simulink library "Nibble_Multiplexers_Lib"  (R2023a)
settings: Solver=ode45  StartTime=0.0  StopTime=10.0  RelTol=1e-3  EnableMultiTasking=on
settings Model: Creator=uzivatel  LastModifiedBy=Jozko Mrkvicka
settings SolverCC: AlgebraicLoopSolver=TrustRegion
settings DataIOCC: LimitDataPoints=on  SaveFormat=Array  ReturnWorkspaceOutputs=off
settings OptimizationCC: LifeSpan=inf
settings DebuggingCC: UnderspecifiedInitializationDetection=Classic  MergeDetectMultiDrivingBlocksExec=none  SolverPrmCheckMsg=warning  UnconnectedInputMsg=warning  UnconnectedOutputMsg=warning  UnconnectedLineMsg=warning  StateNameClashWarn=warning  SFUnexpectedBacktrackingDiag=warning  SFNoUnconditionalDefaultTransitionDiag=warning  ArithmeticOperatorsInVariantConditions=warning
settings HardwareCC: ProdBitPerPointer=32  ProdBitPerSizeT=32  ProdBitPerPtrDiffT=32  ProdLargestAtomicFloat=None  ProdIntDivRoundTo=Undefined  ProdEndianess=Unspecified  ProdWordSize=32  ProdHWDeviceType=32-bit Generic
settings ModelReferenceCC: EnableRefExpFcnMdlSchedulingChecks=on  PropagateSignalLabelsOutOfModel=off
settings SFSimCC: SimUseLocalCustomCode=off  CustomCodeUndefinedFunction=UseInterfaceOnly
settings RTWCC: RTWUseLocalCustomCode=off
settings CodeAppCC: StateflowObjectComments=on
settings GRTTargetCC: TargetLangStandard=C89/C90 (ANSI)
settings ConfigComp: CovMetricSettings=dw  CovSaveCumulativeToWorkspaceVar=on  CovSaveSingleToWorkspaceVar=on  CovExternalEMLEnable=off

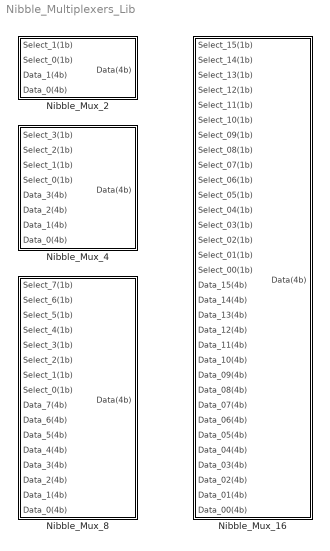
== system Nibble_Multiplexers_Lib ==
  Nibble_Mux_16 : Subsystem
  Nibble_Mux_2 : Subsystem
  Nibble_Mux_4 : Subsystem
  Nibble_Mux_8 : Subsystem

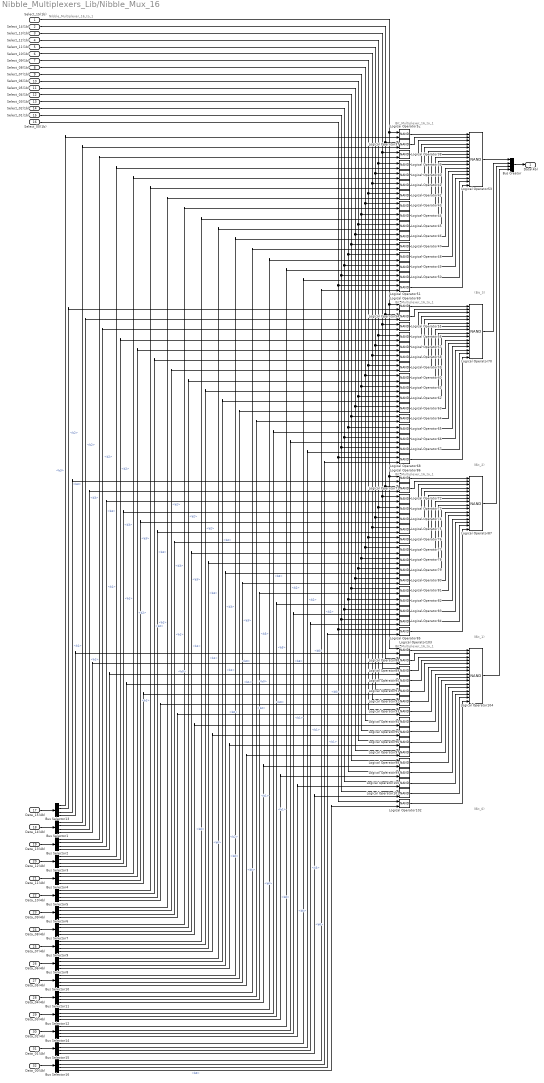
== system Nibble_Multiplexers_Lib/Nibble_Mux_16 ==
  note: (Bit_3)
  note: (Bit_2)
  note: Bit_Multiplexer_16_to_1
  note: (Bit_1)
  note: Bit_Multiplexer_16_to_1
  note: (Bit_0)
  note: Bit_Multiplexer_16_to_1
  note: Bit_Multiplexer_16_to_1
  note: Nibble_Multiplexer_16_to_1
  Select_15(1b) : Inport
  Select_14(1b) : Inport  Port=2
  Select_13(1b) : Inport  Port=3
  Select_12(1b) : Inport  Port=4
  Select_11(1b) : Inport  Port=5
  Select_10(1b) : Inport  Port=6
  Select_09(1b) : Inport  Port=7
  Select_08(1b) : Inport  Port=8
  Select_07(1b) : Inport  Port=9
  Select_06(1b) : Inport  Port=10
  Select_05(1b) : Inport  Port=11
  Select_04(1b) : Inport  Port=12
  Select_03(1b) : Inport  Port=13
  Select_02(1b) : Inport  Port=14
  Select_01(1b) : Inport  Port=15
  Select_00(1b) : Inport  Port=16
  Data_15(4b) : Inport  Port=17
  Data_14(4b) : Inport  Port=18
  Data_13(4b) : Inport  Port=19
  Data_12(4b) : Inport  Port=20
  Data_11(4b) : Inport  Port=21
  Data_10(4b) : Inport  Port=22
  Data_09(4b) : Inport  Port=23
  Data_08(4b) : Inport  Port=24
  Data_07(4b) : Inport  Port=25
  Data_06(4b) : Inport  Port=26
  Data_05(4b) : Inport  Port=27
  Data_04(4b) : Inport  Port=28
  Data_03(4b) : Inport  Port=29
  Data_02(4b) : Inport  Port=30
  Data_01(4b) : Inport  Port=31
  Data_00(4b) : Inport  Port=32
  Bus Creator : BusCreator  Inputs=4
  Bus Selector{1..16} (16 alike) : BusSelector  OutputSignals=b3,b2,b1,b0
  Logical Operator{37..52,54..69,71..86,88..103} (64 alike) : Logic  Operator=NAND  IconShape=distinctive  AllPortsSameDT=off  OutDataTypeStr=boolean
  Logical Operator{53,70,87,104} (4 alike) : Logic  Operator=NAND  Inputs=16  IconShape=distinctive  OutDataTypeStr=boolean
  Data(4b) : Outport
  wires:
  Bus Selector13/1 -> Logical Operator52/2  "<b3>"
  Bus Selector1/1 -> Logical Operator37/2  "<b3>"
  Bus Selector2/1 -> Logical Operator38/2  "<b3>"
  Bus Selector3/1 -> Logical Operator39/2  "<b3>"
  Bus Selector4/1 -> Logical Operator40/2  "<b3>"
  Bus Selector5/1 -> Logical Operator41/2  "<b3>"
  Bus Selector6/1 -> Logical Operator42/2  "<b3>"
  Bus Selector7/1 -> Logical Operator43/2  "<b3>"
  Bus Selector13/2 -> Logical Operator69/2  "<b2>"
  Bus Selector1/2 -> Logical Operator54/2  "<b2>"
  Bus Selector2/2 -> Logical Operator55/2  "<b2>"
  Bus Selector3/2 -> Logical Operator56/2  "<b2>"
  Bus Selector4/2 -> Logical Operator57/2  "<b2>"
  Bus Selector5/2 -> Logical Operator58/2  "<b2>"
  Bus Selector6/2 -> Logical Operator59/2  "<b2>"
  Bus Selector7/2 -> Logical Operator60/2  "<b2>"
  Bus Selector13/3 -> Logical Operator86/2  "<b1>"
  Bus Selector1/3 -> Logical Operator71/2  "<b1>"
  Bus Selector2/3 -> Logical Operator72/2  "<b1>"
  Bus Selector3/3 -> Logical Operator73/2  "<b1>"
  Bus Selector4/3 -> Logical Operator74/2  "<b1>"
  Bus Selector5/3 -> Logical Operator75/2  "<b1>"
  Bus Selector6/3 -> Logical Operator76/2  "<b1>"
  Bus Selector7/3 -> Logical Operator77/2  "<b1>"
  Bus Selector13/4 -> Logical Operator103/2  "<b0>"
  Bus Selector1/4 -> Logical Operator88/2  "<b0>"
  Bus Selector2/4 -> Logical Operator89/2  "<b0>"
  Bus Selector3/4 -> Logical Operator90/2  "<b0>"
  Bus Selector4/4 -> Logical Operator91/2  "<b0>"
  Bus Selector5/4 -> Logical Operator92/2  "<b0>"
  Bus Selector6/4 -> Logical Operator93/2  "<b0>"
  Bus Selector7/4 -> Logical Operator94/2  "<b0>"
  Logical Operator49/1 -> Logical Operator53/14
  Logical Operator43/1 -> Logical Operator53/8
  Logical Operator51/1 -> Logical Operator53/16
  Logical Operator46/1 -> Logical Operator53/11
  Logical Operator50/1 -> Logical Operator53/15
  Logical Operator37/1 -> Logical Operator53/2
  Logical Operator47/1 -> Logical Operator53/12
  Logical Operator39/1 -> Logical Operator53/4
  Logical Operator38/1 -> Logical Operator53/3
  Logical Operator44/1 -> Logical Operator53/9
  Logical Operator45/1 -> Logical Operator53/10
  Logical Operator40/1 -> Logical Operator53/5
  Logical Operator52/1 -> Logical Operator53/1
  Logical Operator42/1 -> Logical Operator53/7
  Logical Operator41/1 -> Logical Operator53/6
  Logical Operator48/1 -> Logical Operator53/13
  Logical Operator66/1 -> Logical Operator70/14
  Logical Operator60/1 -> Logical Operator70/8
  Logical Operator68/1 -> Logical Operator70/16
  Logical Operator63/1 -> Logical Operator70/11
  Logical Operator67/1 -> Logical Operator70/15
  Logical Operator54/1 -> Logical Operator70/2
  Logical Operator64/1 -> Logical Operator70/12
  Logical Operator56/1 -> Logical Operator70/4
  Logical Operator55/1 -> Logical Operator70/3
  Logical Operator61/1 -> Logical Operator70/9
  Logical Operator62/1 -> Logical Operator70/10
  Logical Operator57/1 -> Logical Operator70/5
  Logical Operator69/1 -> Logical Operator70/1
  Logical Operator59/1 -> Logical Operator70/7
  Logical Operator58/1 -> Logical Operator70/6
  Logical Operator65/1 -> Logical Operator70/13
  Logical Operator83/1 -> Logical Operator87/14
  Logical Operator77/1 -> Logical Operator87/8
  Logical Operator85/1 -> Logical Operator87/16
  Logical Operator80/1 -> Logical Operator87/11
  Logical Operator84/1 -> Logical Operator87/15
  Logical Operator71/1 -> Logical Operator87/2
  Logical Operator81/1 -> Logical Operator87/12
  Logical Operator73/1 -> Logical Operator87/4
  Logical Operator72/1 -> Logical Operator87/3
  Logical Operator78/1 -> Logical Operator87/9
  Logical Operator79/1 -> Logical Operator87/10
  Logical Operator74/1 -> Logical Operator87/5
  Logical Operator86/1 -> Logical Operator87/1
  Logical Operator76/1 -> Logical Operator87/7
  Logical Operator75/1 -> Logical Operator87/6
  Logical Operator82/1 -> Logical Operator87/13
  Logical Operator100/1 -> Logical Operator104/14
  Logical Operator94/1 -> Logical Operator104/8
  Logical Operator102/1 -> Logical Operator104/16
  Logical Operator97/1 -> Logical Operator104/11
  Logical Operator101/1 -> Logical Operator104/15
  Logical Operator88/1 -> Logical Operator104/2
  Logical Operator98/1 -> Logical Operator104/12
  Logical Operator90/1 -> Logical Operator104/4
  Logical Operator89/1 -> Logical Operator104/3
  Logical Operator95/1 -> Logical Operator104/9
  Logical Operator96/1 -> Logical Operator104/10
  Logical Operator91/1 -> Logical Operator104/5
  Logical Operator103/1 -> Logical Operator104/1
  Logical Operator93/1 -> Logical Operator104/7
  Logical Operator92/1 -> Logical Operator104/6
  Logical Operator99/1 -> Logical Operator104/13
  Logical Operator53/1 -> Bus Creator/1
  Logical Operator104/1 -> Bus Creator/4
  Logical Operator87/1 -> Bus Creator/3
  Logical Operator70/1 -> Bus Creator/2
  Bus Creator/1 -> Data(4b)/1
  Select_15(1b)/1 -> Logical Operator52/1, Logical Operator86/1, Logical Operator103/1, Logical Operator69/1
  Select_14(1b)/1 -> Logical Operator37/1, Logical Operator71/1, Logical Operator88/1, Logical Operator54/1
  Select_13(1b)/1 -> Logical Operator38/1, Logical Operator72/1, Logical Operator89/1, Logical Operator55/1
  Select_12(1b)/1 -> Logical Operator39/1, Logical Operator73/1, Logical Operator90/1, Logical Operator56/1
  Select_11(1b)/1 -> Logical Operator40/1, Logical Operator74/1, Logical Operator91/1, Logical Operator57/1
  Select_10(1b)/1 -> Logical Operator41/1, Logical Operator75/1, Logical Operator92/1, Logical Operator58/1
  Select_09(1b)/1 -> Logical Operator42/1, Logical Operator76/1, Logical Operator93/1, Logical Operator59/1
  Select_08(1b)/1 -> Logical Operator43/1, Logical Operator77/1, Logical Operator94/1, Logical Operator60/1
  Select_07(1b)/1 -> Logical Operator44/1, Logical Operator78/1, Logical Operator95/1, Logical Operator61/1
  Select_04(1b)/1 -> Logical Operator47/1, Logical Operator81/1, Logical Operator98/1, Logical Operator64/1
  Select_03(1b)/1 -> Logical Operator48/1, Logical Operator82/1, Logical Operator99/1, Logical Operator65/1
  Select_01(1b)/1 -> Logical Operator50/1, Logical Operator84/1, Logical Operator101/1, Logical Operator67/1
  Select_00(1b)/1 -> Logical Operator51/1, Logical Operator85/1, Logical Operator102/1, Logical Operator68/1
  Select_06(1b)/1 -> Logical Operator45/1, Logical Operator79/1, Logical Operator96/1, Logical Operator62/1
  Select_05(1b)/1 -> Logical Operator46/1, Logical Operator80/1, Logical Operator97/1, Logical Operator63/1
  Select_02(1b)/1 -> Logical Operator49/1, Logical Operator83/1, Logical Operator100/1, Logical Operator66/1
  Bus Selector9/1 -> Logical Operator44/2  "<b3>"
  Bus Selector9/2 -> Logical Operator61/2  "<b2>"
  Bus Selector9/3 -> Logical Operator78/2  "<b1>"
  Bus Selector9/4 -> Logical Operator95/2  "<b0>"
  Bus Selector8/1 -> Logical Operator45/2  "<b3>"
  Bus Selector8/2 -> Logical Operator62/2  "<b2>"
  Bus Selector8/3 -> Logical Operator79/2  "<b1>"
  Bus Selector8/4 -> Logical Operator96/2  "<b0>"
  Bus Selector10/1 -> Logical Operator46/2  "<b3>"
  Bus Selector10/2 -> Logical Operator63/2  "<b2>"
  Bus Selector10/3 -> Logical Operator80/2  "<b1>"
  Bus Selector10/4 -> Logical Operator97/2  "<b0>"
  Bus Selector11/1 -> Logical Operator47/2  "<b3>"
  Bus Selector11/2 -> Logical Operator64/2  "<b2>"
  Bus Selector11/4 -> Logical Operator98/2  "<b0>"
  Bus Selector11/3 -> Logical Operator81/2  "<b1>"
  Bus Selector12/1 -> Logical Operator48/2  "<b3>"
  Bus Selector12/2 -> Logical Operator65/2  "<b2>"
  Bus Selector12/3 -> Logical Operator82/2  "<b1>"
  Bus Selector12/4 -> Logical Operator99/2  "<b0>"
  Bus Selector14/1 -> Logical Operator49/2  "<b3>"
  Bus Selector14/2 -> Logical Operator66/2  "<b2>"
  Bus Selector14/3 -> Logical Operator83/2  "<b1>"
  Bus Selector14/4 -> Logical Operator100/2  "<b0>"
  Bus Selector15/1 -> Logical Operator50/2  "<b3>"
  Bus Selector15/2 -> Logical Operator67/2  "<b2>"
  Bus Selector15/3 -> Logical Operator84/2  "<b1>"
  Bus Selector15/4 -> Logical Operator101/2  "<b0>"
  Bus Selector16/1 -> Logical Operator51/2  "<b3>"
  Bus Selector16/2 -> Logical Operator68/2  "<b2>"
  Bus Selector16/3 -> Logical Operator85/2  "<b1>"
  Bus Selector16/4 -> Logical Operator102/2  "<b0>"
  Data_15(4b)/1 -> Bus Selector13/1
  Data_14(4b)/1 -> Bus Selector1/1
  Data_13(4b)/1 -> Bus Selector2/1
  Data_12(4b)/1 -> Bus Selector3/1
  Data_11(4b)/1 -> Bus Selector4/1
  Data_10(4b)/1 -> Bus Selector5/1
  Data_09(4b)/1 -> Bus Selector6/1
  Data_08(4b)/1 -> Bus Selector7/1
  Data_07(4b)/1 -> Bus Selector9/1
  Data_06(4b)/1 -> Bus Selector8/1
  Data_05(4b)/1 -> Bus Selector10/1
  Data_04(4b)/1 -> Bus Selector11/1
  Data_03(4b)/1 -> Bus Selector12/1
  Data_02(4b)/1 -> Bus Selector14/1
  Data_01(4b)/1 -> Bus Selector15/1
  Data_00(4b)/1 -> Bus Selector16/1

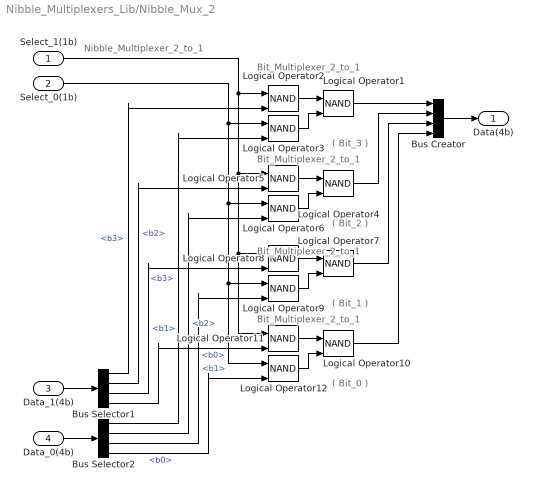
== system Nibble_Multiplexers_Lib/Nibble_Mux_2 ==
  note: Nibble_Multiplexer_2_to_1
  note: Bit_Multiplexer_2_to_1
  note: ( Bit_3 )
  note: Bit_Multiplexer_2_to_1
  note: ( Bit_2 )
  note: Bit_Multiplexer_2_to_1
  note: ( Bit_1 )
  note: Bit_Multiplexer_2_to_1
  note: ( Bit_0 )
  Select_1(1b) : Inport
  Select_0(1b) : Inport  Port=2
  Data_1(4b) : Inport  Port=3
  Data_0(4b) : Inport  Port=4
  Bus Creator : BusCreator  Inputs=4
  Bus Selector1 : BusSelector  OutputSignals=b3,b2,b1,b0
  Bus Selector2 : BusSelector  OutputSignals=b3,b2,b1,b0
  Logical Operator{1..12} (12 alike) : Logic  Operator=NAND  IconShape=distinctive  AllPortsSameDT=off  OutDataTypeStr=boolean
  Data(4b) : Outport
  wires:
  Data_0(4b)/1 -> Bus Selector2/1
  Bus Selector2/4 -> Logical Operator12/2  "<b0>"
  Bus Selector1/4 -> Logical Operator11/2  "<b0>"
  Bus Selector1/3 -> Logical Operator8/2  "<b1>"
  Bus Selector2/3 -> Logical Operator9/2  "<b1>"
  Bus Selector1/2 -> Logical Operator5/2  "<b2>"
  Bus Selector2/2 -> Logical Operator6/2  "<b2>"
  Bus Selector2/1 -> Logical Operator3/2  "<b3>"
  Bus Selector1/1 -> Logical Operator2/2  "<b3>"
  Select_0(1b)/1 -> Logical Operator3/1, Logical Operator6/1, Logical Operator12/1, Logical Operator9/1
  Select_1(1b)/1 -> Logical Operator2/1, Logical Operator5/1, Logical Operator11/1, Logical Operator8/1
  Logical Operator3/1 -> Logical Operator1/2
  Logical Operator2/1 -> Logical Operator1/1
  Logical Operator6/1 -> Logical Operator4/2
  Logical Operator5/1 -> Logical Operator4/1
  Logical Operator9/1 -> Logical Operator7/2
  Logical Operator8/1 -> Logical Operator7/1
  Logical Operator12/1 -> Logical Operator10/2
  Logical Operator11/1 -> Logical Operator10/1
  Bus Creator/1 -> Data(4b)/1
  Data_1(4b)/1 -> Bus Selector1/1
  Logical Operator1/1 -> Bus Creator/1
  Logical Operator4/1 -> Bus Creator/2
  Logical Operator7/1 -> Bus Creator/3
  Logical Operator10/1 -> Bus Creator/4

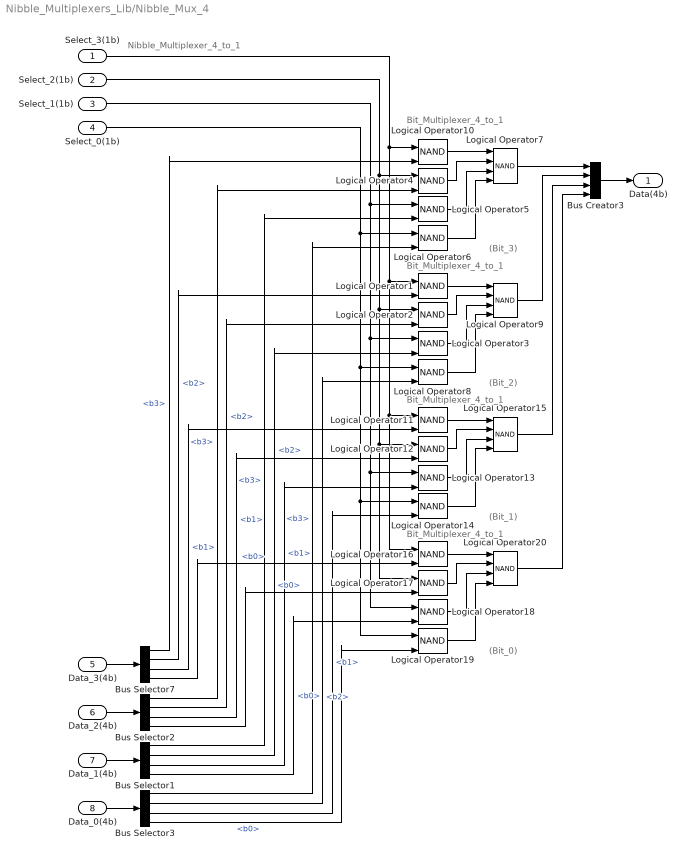
== system Nibble_Multiplexers_Lib/Nibble_Mux_4 ==
  note: Nibble_Multiplexer_4_to_1
  note: Bit_Multiplexer_4_to_1
  note: (Bit_3)
  note: Bit_Multiplexer_4_to_1
  note: (Bit_2)
  note: Bit_Multiplexer_4_to_1
  note: (Bit_1)
  note: Bit_Multiplexer_4_to_1
  note: (Bit_0)
  Select_3(1b) : Inport
  Select_2(1b) : Inport  Port=2
  Select_1(1b) : Inport  Port=3
  Select_0(1b) : Inport  Port=4
  Data_3(4b) : Inport  Port=5
  Data_2(4b) : Inport  Port=6
  Data_1(4b) : Inport  Port=7
  Data_0(4b) : Inport  Port=8
  Bus Creator3 : BusCreator  Inputs=4
  Bus Selector{1..3,7} (4 alike) : BusSelector  OutputSignals=b3,b2,b1,b0
  Logical Operator{1..6,8,10..14,16..19} (16 alike) : Logic  Operator=NAND  IconShape=distinctive  AllPortsSameDT=off  OutDataTypeStr=boolean
  Logical Operator{7,9,15,20} (4 alike) : Logic  Operator=NAND  Inputs=4  IconShape=distinctive  OutDataTypeStr=boolean
  Data(4b) : Outport
  wires:
  Bus Creator3/1 -> Data(4b)/1
  Logical Operator20/1 -> Bus Creator3/4
  Logical Operator15/1 -> Bus Creator3/3
  Logical Operator9/1 -> Bus Creator3/2
  Logical Operator7/1 -> Bus Creator3/1
  Bus Selector7/4 -> Logical Operator16/2  "<b0>"
  Bus Selector2/4 -> Logical Operator17/2  "<b0>"
  Bus Selector1/4 -> Logical Operator18/2  "<b0>"
  Bus Selector3/4 -> Logical Operator19/2  "<b0>"
  Bus Selector7/3 -> Logical Operator11/2  "<b1>"
  Bus Selector2/3 -> Logical Operator12/2  "<b1>"
  Bus Selector1/3 -> Logical Operator13/2  "<b1>"
  Bus Selector3/3 -> Logical Operator14/2  "<b1>"
  Bus Selector7/2 -> Logical Operator1/2  "<b2>"
  Bus Selector2/2 -> Logical Operator2/2  "<b2>"
  Bus Selector1/2 -> Logical Operator3/2  "<b2>"
  Bus Selector3/2 -> Logical Operator8/2  "<b2>"
  Bus Selector7/1 -> Logical Operator10/2  "<b3>"
  Bus Selector2/1 -> Logical Operator4/2  "<b3>"
  Bus Selector1/1 -> Logical Operator5/2  "<b3>"
  Bus Selector3/1 -> Logical Operator6/2  "<b3>"
  Select_0(1b)/1 -> Logical Operator6/1, Logical Operator8/1, Logical Operator19/1, Logical Operator14/1
  Select_1(1b)/1 -> Logical Operator5/1, Logical Operator3/1, Logical Operator18/1, Logical Operator13/1
  Select_2(1b)/1 -> Logical Operator17/1, Logical Operator12/1, Logical Operator2/1, Logical Operator4/1
  Select_3(1b)/1 -> Logical Operator10/1, Logical Operator16/1, Logical Operator11/1, Logical Operator1/1
  Data_3(4b)/1 -> Bus Selector7/1
  Data_2(4b)/1 -> Bus Selector2/1
  Data_1(4b)/1 -> Bus Selector1/1
  Data_0(4b)/1 -> Bus Selector3/1
  Logical Operator6/1 -> Logical Operator7/4
  Logical Operator10/1 -> Logical Operator7/1
  Logical Operator4/1 -> Logical Operator7/2
  Logical Operator5/1 -> Logical Operator7/3
  Logical Operator8/1 -> Logical Operator9/4
  Logical Operator1/1 -> Logical Operator9/1
  Logical Operator2/1 -> Logical Operator9/2
  Logical Operator3/1 -> Logical Operator9/3
  Logical Operator14/1 -> Logical Operator15/4
  Logical Operator11/1 -> Logical Operator15/1
  Logical Operator12/1 -> Logical Operator15/2
  Logical Operator13/1 -> Logical Operator15/3
  Logical Operator19/1 -> Logical Operator20/4
  Logical Operator16/1 -> Logical Operator20/1
  Logical Operator17/1 -> Logical Operator20/2
  Logical Operator18/1 -> Logical Operator20/3

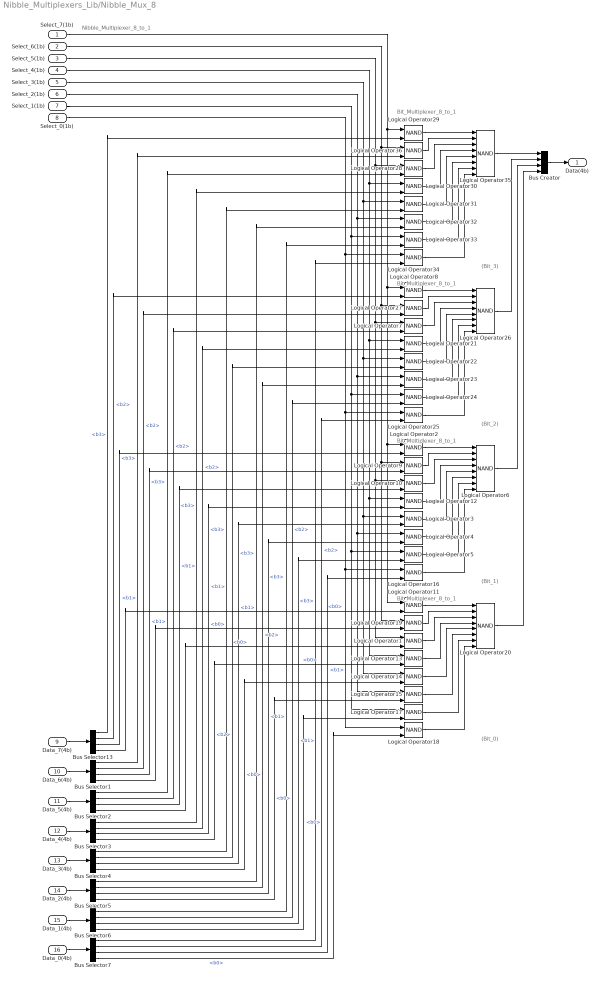
== system Nibble_Multiplexers_Lib/Nibble_Mux_8 ==
  note: Nibble_Multiplexer_8_to_1
  note: Bit_Multiplexer_8_to_1
  note: (Bit_2)
  note: (Bit_3)
  note: (Bit_0)
  note: Bit_Multiplexer_8_to_1
  note: Bit_Multiplexer_8_to_1
  note: (Bit_1)
  note: Bit_Multiplexer_8_to_1
  Select_7(1b) : Inport
  Select_6(1b) : Inport  Port=2
  Select_5(1b) : Inport  Port=3
  Select_4(1b) : Inport  Port=4
  Select_3(1b) : Inport  Port=5
  Select_2(1b) : Inport  Port=6
  Select_1(1b) : Inport  Port=7
  Select_0(1b) : Inport  Port=8
  Data_7(4b) : Inport  Port=9
  Data_6(4b) : Inport  Port=10
  Data_5(4b) : Inport  Port=11
  Data_4(4b) : Inport  Port=12
  Data_3(4b) : Inport  Port=13
  Data_2(4b) : Inport  Port=14
  Data_1(4b) : Inport  Port=15
  Data_0(4b) : Inport  Port=16
  Bus Creator : BusCreator  Inputs=4
  Bus Selector{1..7,13} (8 alike) : BusSelector  OutputSignals=b3,b2,b1,b0
  Logical Operator{1..5,7..19,21..25,27..34,36} (32 alike) : Logic  Operator=NAND  IconShape=distinctive  AllPortsSameDT=off  OutDataTypeStr=boolean
  Logical Operator{6,20,26,35} (4 alike) : Logic  Operator=NAND  Inputs=8  IconShape=distinctive  OutDataTypeStr=boolean
  Data(4b) : Outport
  wires:
  Bus Creator/1 -> Data(4b)/1
  Bus Selector13/1 -> Logical Operator29/2  "<b3>"
  Bus Selector1/1 -> Logical Operator36/2  "<b3>"
  Bus Selector2/1 -> Logical Operator28/2  "<b3>"
  Bus Selector3/1 -> Logical Operator30/2  "<b3>"
  Bus Selector4/1 -> Logical Operator31/2  "<b3>"
  Bus Selector5/1 -> Logical Operator32/2  "<b3>"
  Bus Selector6/1 -> Logical Operator33/2  "<b3>"
  Bus Selector7/1 -> Logical Operator34/2  "<b3>"
  Bus Selector13/2 -> Logical Operator8/2  "<b2>"
  Bus Selector1/2 -> Logical Operator27/2  "<b2>"
  Bus Selector2/2 -> Logical Operator7/2  "<b2>"
  Bus Selector3/2 -> Logical Operator21/2  "<b2>"
  Bus Selector4/2 -> Logical Operator22/2  "<b2>"
  Bus Selector5/2 -> Logical Operator23/2  "<b2>"
  Bus Selector6/2 -> Logical Operator24/2  "<b2>"
  Bus Selector7/2 -> Logical Operator25/2  "<b2>"
  Bus Selector13/3 -> Logical Operator2/2  "<b1>"
  Bus Selector1/3 -> Logical Operator9/2  "<b1>"
  Bus Selector2/3 -> Logical Operator10/2  "<b1>"
  Bus Selector3/3 -> Logical Operator12/2  "<b1>"
  Bus Selector4/3 -> Logical Operator3/2  "<b1>"
  Bus Selector5/3 -> Logical Operator4/2  "<b1>"
  Bus Selector6/3 -> Logical Operator5/2  "<b1>"
  Bus Selector7/3 -> Logical Operator16/2  "<b1>"
  Bus Selector13/4 -> Logical Operator11/2  "<b0>"
  Bus Selector1/4 -> Logical Operator19/2  "<b0>"
  Bus Selector2/4 -> Logical Operator1/2  "<b0>"
  Bus Selector3/4 -> Logical Operator13/2  "<b0>"
  Bus Selector4/4 -> Logical Operator14/2  "<b0>"
  Bus Selector5/4 -> Logical Operator15/2  "<b0>"
  Bus Selector6/4 -> Logical Operator17/2  "<b0>"
  Bus Selector7/4 -> Logical Operator18/2  "<b0>"
  Data_7(4b)/1 -> Bus Selector13/1
  Data_6(4b)/1 -> Bus Selector1/1
  Data_0(4b)/1 -> Bus Selector7/1
  Data_1(4b)/1 -> Bus Selector6/1
  Data_2(4b)/1 -> Bus Selector5/1
  Data_3(4b)/1 -> Bus Selector4/1
  Data_4(4b)/1 -> Bus Selector3/1
  Data_5(4b)/1 -> Bus Selector2/1
  Select_7(1b)/1 -> Logical Operator11/1, Logical Operator2/1, Logical Operator8/1, Logical Operator29/1
  Select_6(1b)/1 -> Logical Operator19/1, Logical Operator9/1, Logical Operator27/1, Logical Operator36/1
  Select_5(1b)/1 -> Logical Operator28/1, Logical Operator7/1, Logical Operator10/1, Logical Operator1/1
  Select_4(1b)/1 -> Logical Operator30/1, Logical Operator21/1, Logical Operator12/1, Logical Operator13/1
  Select_3(1b)/1 -> Logical Operator31/1, Logical Operator22/1, Logical Operator3/1, Logical Operator14/1
  Select_2(1b)/1 -> Logical Operator32/1, Logical Operator23/1, Logical Operator4/1, Logical Operator15/1
  Select_1(1b)/1 -> Logical Operator33/1, Logical Operator24/1, Logical Operator5/1, Logical Operator17/1
  Select_0(1b)/1 -> Logical Operator34/1, Logical Operator25/1, Logical Operator16/1, Logical Operator18/1
  Logical Operator25/1 -> Logical Operator26/8
  Logical Operator24/1 -> Logical Operator26/7
  Logical Operator23/1 -> Logical Operator26/6
  Logical Operator21/1 -> Logical Operator26/4
  Logical Operator7/1 -> Logical Operator26/3
  Logical Operator27/1 -> Logical Operator26/2
  Logical Operator6/1 -> Bus Creator/3
  Logical Operator33/1 -> Logical Operator35/7
  Logical Operator36/1 -> Logical Operator35/2
  Logical Operator29/1 -> Logical Operator35/1
  Logical Operator28/1 -> Logical Operator35/3
  Logical Operator34/1 -> Logical Operator35/8
  Logical Operator31/1 -> Logical Operator35/5
  Logical Operator30/1 -> Logical Operator35/4
  Logical Operator32/1 -> Logical Operator35/6
  Logical Operator20/1 -> Bus Creator/4
  Logical Operator17/1 -> Logical Operator20/7
  Logical Operator35/1 -> Bus Creator/1
  Logical Operator18/1 -> Logical Operator20/8
  Logical Operator1/1 -> Logical Operator20/3
  Logical Operator19/1 -> Logical Operator20/2
  Logical Operator15/1 -> Logical Operator20/6
  Logical Operator26/1 -> Bus Creator/2
  Logical Operator5/1 -> Logical Operator6/7
  Logical Operator22/1 -> Logical Operator26/5
  Logical Operator2/1 -> Logical Operator6/1
  Logical Operator13/1 -> Logical Operator20/4
  Logical Operator3/1 -> Logical Operator6/5
  Logical Operator12/1 -> Logical Operator6/4
  Logical Operator9/1 -> Logical Operator6/2
  Logical Operator16/1 -> Logical Operator6/8
  Logical Operator4/1 -> Logical Operator6/6
  Logical Operator14/1 -> Logical Operator20/5
  Logical Operator8/1 -> Logical Operator26/1
  Logical Operator10/1 -> Logical Operator6/3
  Logical Operator11/1 -> Logical Operator20/1
